simulink model "simulation_model"  (R2025a)
settings: Solver=ode4  StartTime=0.0  StopTime=1500  FixedStep=0.5  RelTol=1e-3
InitFcn:
  | init
StopFcn:
  | post_processing
values from neighbouring files (symbols this model uses):
  A0 = deg2rad(A0)    [init.m]
  delta0 = deg2rad(delta0)    [init.m]
  dT = 10    [init.m]
  fc = 0.62    [init.m]
  g = 9.80665    [init.m]
  Isp = zeros(1, 3)    [init.m]
  l_trilho = lt    (= 20.71)    [init.m]
  lc = 1.4    [init.m]
  lon0 = deg2rad(lon0)    [init.m]
  m0 = sum(mp) + sum(ms) + mL    [init.m]
  mp = zeros(1, 3)    [init.m]
  ms = zeros(1, 3)    [init.m]
  parametros_aero = [ts, Sr, fc]    [init.m]
  parametros_grav = [Re,mut,J2,J3,J4]    [init.m]
  phi0 = deg2rad(phi0)    [init.m]
  r0 = Re + h0    (= 6378137)    [init.m]
  Re = 6378.1370e3    (= 6378137)    [init.m]
  Sr = [S1, S2 * f2, S3 * f3, SL * f4]    [init.m]
  ti = zeros(1, 3)    [init.m]
  tq = zeros(1, 3)    [init.m]
  ts = zeros(1, 3)    [init.m]
  V0 = 7.2921150e-5    (= 7.292115e-05)    [init.m]
  we = 7.2921150e-5    (= 7.292115e-05)    [init.m]
settings Model: Creator=Guilherme  LastModifiedBy=Guilherme

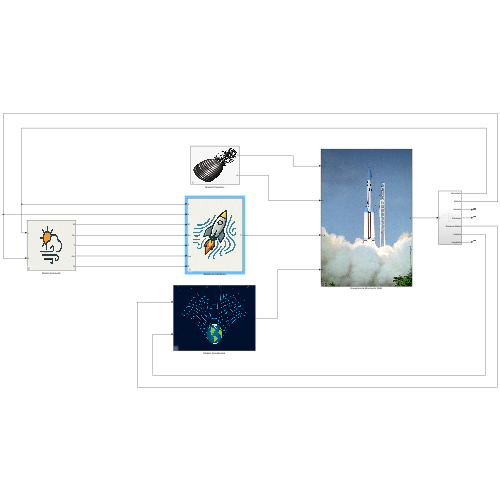
[thumbnail: Simulink's stored preview of the top-level diagram]
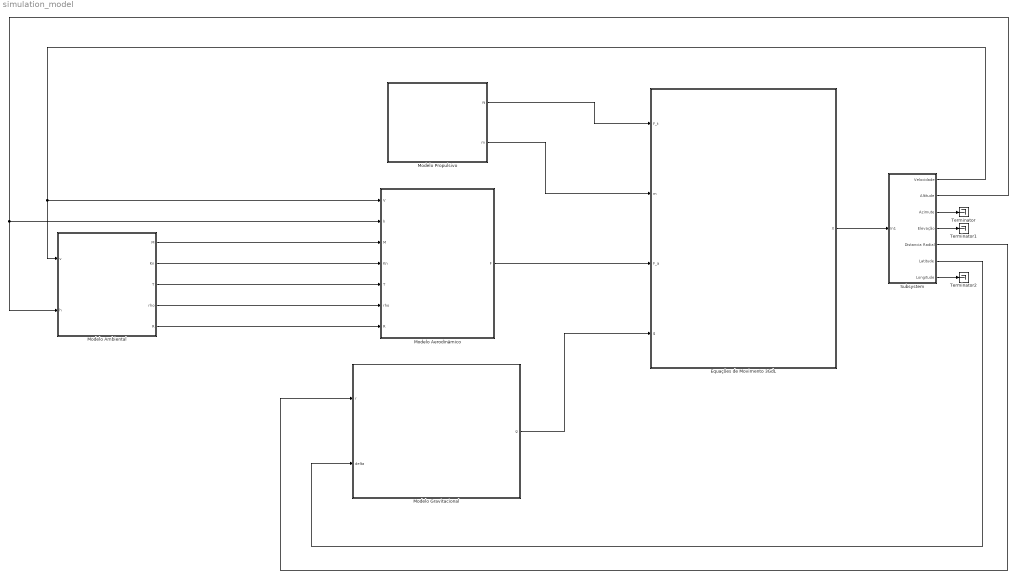
== system simulation_model ==
  Equações de Movimento 3GdL : Subsystem  mask{estado_inicial=[V0; A0; phi0; r0; delta0; lon0], trilho=l_trilho}
      mask prompts: estado_inicial "Vetor de estados inicial:"; trilho "Comprimeto do trilho de lançameto:"
      mask DialogControl texto Prompt: Bloco utilizado para simular as equações de movimento 3GdL de um foguete com 3 estágios. Os estados são organizados da seguinte forma:
      mask DialogControl Control2 Prompt: ● Magnitude da Velocidade - [m/s];
      mask DialogControl Control3 Prompt: ● Azimute Relativo - [rad];
      mask DialogControl Control4 Prompt: ● Ângulo de elevação da velocidade relativa - [rad];
      mask DialogControl Control5 Prompt: ● Distancia radial - [m];
      mask DialogControl Control6 Prompt: ● Latitude planetária - [rad];
      mask DialogControl Control7 Prompt: ● Longitude planetária - [rad].
      mask Display: image('EoM_mask.png');
  Modelo Aerodinâmico : Subsystem  mask{t_sep=ts, S_ref=Sr, fator_arrasto=fc}
      mask prompts: t_sep "Instante de separação dos estágios:"; S_ref "Vetor de áreas de referência:"; fator_arrasto "Fator de correção do arrasto:"
      mask DialogControl Control1 Prompt: Bloco utilizado para modelar a aerodinâmica do foguete. Calcula a força de arrasto a partir da velocidade e dos parâmetros atmosféricos. Os ângulos de ataque e derrapagem são assumidos zero.
      mask Display: image('aerodinamica_mask.png');
  Modelo Ambiental : Subsystem  mask{comprimento=lc, delta_T=dT}
      mask prompts: comprimento "Comprimento característico do veículo:"; delta_T "Variação de temperatura em relação à atmosfera padrão (15ºC no nível do mar):"
      mask DialogControl Control1 Prompt: Bloco utilizado para implementar o modelo de atmosfera padrão. Calcula os parâmetros atmosféricos com base na altitude de voo e velocidade.
      mask Display: image('atmosfera_mask.png');
  Modelo Gravitacional : Subsystem
      mask DialogControl Control1 Prompt: Bloco utilizado para implementar o modelo gravitacional do planeta Terra. Calcula as componentes centrípeta e radial da gravidade a partir da altitude e latitude do foguete.
      mask Display: image('gravidade_mask.png');
  Modelo Propulsivo : Subsystem  mask{t_ignicao=ti, t_queima=tq, t_sep=ts, massa_prop=mp, massa_est=ms, Isp_sub=Isp, massa0=m0}
      mask prompts: t_ignicao "Instantes de ignição:"; t_queima "Instantes do fim da queima:"; t_sep "Instantes de separação:"; massa_prop "Massa de propelente de cada eságio:"; massa_est "Massa estrutural de cada estágio:"; Isp_sub "Impulso específico de cada estágio:"; massa0 "Massa inicial do foguete:"
      mask DialogControl Control1 Prompt: Bloco utilizado por simular o efeito do sistema propulsivo do foguete. Calcula a força de tração e a massa do veículo a partir do estágio que está operando em cada instante de tempo.
      mask Display: image('motor_mask.jpg');
  Subsystem : Subsystem
  Terminator : Terminator
  Terminator1 : Terminator
  Terminator2 : Terminator
  wires:
  Modelo Propulsivo/1(ft) -> Equações de Movimento 3GdL/1(F_t)
  Modelo Propulsivo/2(m) -> Equações de Movimento 3GdL/2(m)
  Modelo Aerodinâmico/1(F) -> Equações de Movimento 3GdL/3(F_a)
  Modelo Ambiental/1(M) -> Modelo Aerodinâmico/3(M)
  Modelo Ambiental/2(Kn) -> Modelo Aerodinâmico/4(Kn)
  Modelo Ambiental/3(T) -> Modelo Aerodinâmico/5(T)
  Modelo Ambiental/4(rho) -> Modelo Aerodinâmico/6(rho)
  Modelo Ambiental/5(R) -> Modelo Aerodinâmico/7(R)
  Modelo Gravitacional/1(g) -> Equações de Movimento 3GdL/4(g)
  Equações de Movimento 3GdL/1(X) -> Subsystem/1(In1)
  Subsystem/1(Velocidade) -> Modelo Ambiental/1(v), Modelo Aerodinâmico/1(V)
  Subsystem/2(Altitude) -> Modelo Aerodinâmico/2(h), Modelo Ambiental/2(h)
  Subsystem/5(Distancia Radial) -> Modelo Gravitacional/1(r)
  Subsystem/3(Azimute) -> Terminator/1
  Subsystem/4(Elevação) -> Terminator1/1
  Subsystem/7(Longitude) -> Terminator2/1
  Subsystem/6(Latitude) -> Modelo Gravitacional/2(delta)

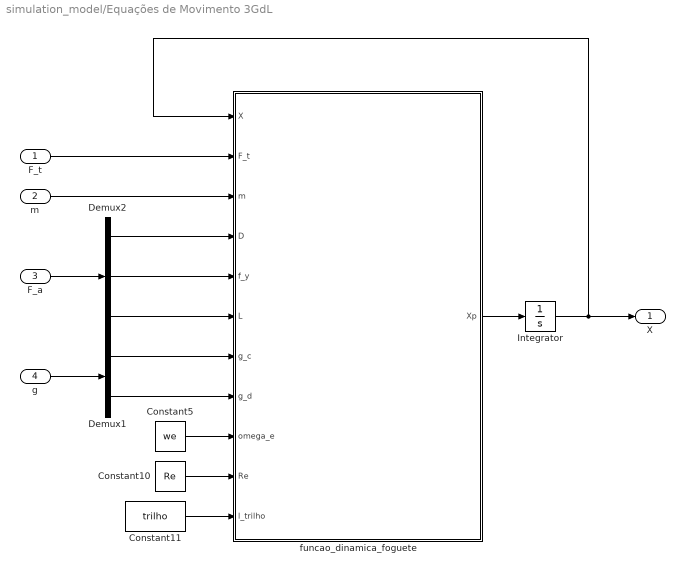
== system simulation_model/Equações de Movimento 3GdL ==
  F_t : Inport
  m : Inport  Port=2
  F_a : Inport  Port=3
  g : Inport  Port=4
  Constant10 : Constant  Value=Re
  Constant11 : Constant  Value=trilho
  Constant5 : Constant  Value=we
  Demux1 : Demux  Outputs=2
  Demux2 : Demux  Outputs=3
  Integrator : Integrator  InitialCondition=estado_inicial
  funcao_dinamica_foguete : MATLAB Function  TreatAsAtomicUnit=on
  X : Outport
  wires:
  Demux2/1 -> funcao_dinamica_foguete/4(D)
  funcao_dinamica_foguete/1(Xp) -> Integrator/1
  Constant5/1 -> funcao_dinamica_foguete/9(omega_e)
  Integrator/1 -> X/1, funcao_dinamica_foguete/1(X)
  Constant10/1 -> funcao_dinamica_foguete/10(Re)
  Demux2/3 -> funcao_dinamica_foguete/6(L)
  F_t/1 -> funcao_dinamica_foguete/2(F_t)
  g/1 -> Demux1/1
  Constant11/1 -> funcao_dinamica_foguete/11(l_trilho)
  Demux1/1 -> funcao_dinamica_foguete/7(g_c)
  Demux2/2 -> funcao_dinamica_foguete/5(f_y)
  Demux1/2 -> funcao_dinamica_foguete/8(g_d)
  m/1 -> funcao_dinamica_foguete/3(m)
  F_a/1 -> Demux2/1

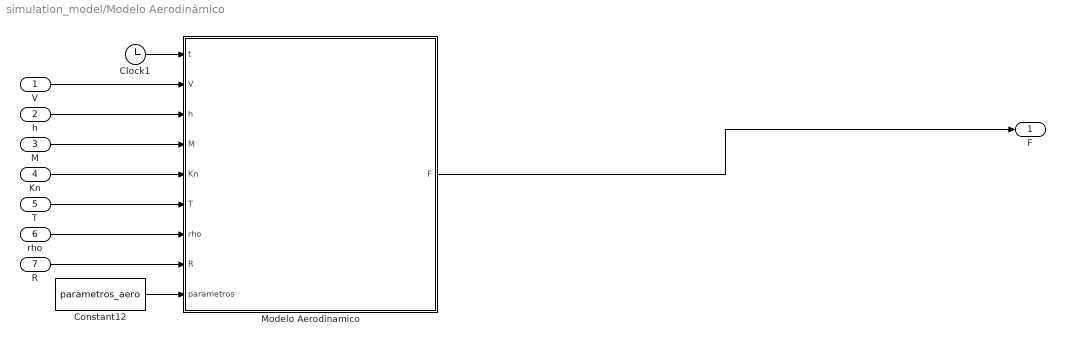
== system simulation_model/Modelo Aerodinâmico ==
  V : Inport
  h : Inport  Port=2
  M : Inport  Port=3
  Kn : Inport  Port=4
  T : Inport  Port=5
  rho : Inport  Port=6
  R : Inport  Port=7
  Clock1 : Clock
  Constant12 : Constant  Value=parametros_aero
  Modelo Aerodinamico : MATLAB Function  TreatAsAtomicUnit=on
  F : Outport
  wires:
  Constant12/1 -> Modelo Aerodinamico/9(parametros)
  M/1 -> Modelo Aerodinamico/4(M)
  Modelo Aerodinamico/1(F) -> F/1
  R/1 -> Modelo Aerodinamico/8(R)
  h/1 -> Modelo Aerodinamico/3(h)
  V/1 -> Modelo Aerodinamico/2(V)
  Clock1/1 -> Modelo Aerodinamico/1(t)
  T/1 -> Modelo Aerodinamico/6(T)
  Kn/1 -> Modelo Aerodinamico/5(Kn)
  rho/1 -> Modelo Aerodinamico/7(rho)

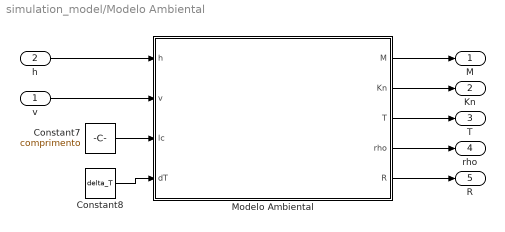
== system simulation_model/Modelo Ambiental ==
  v : Inport
  h : Inport  Port=2
  Constant7 : Constant  Value=comprimento
  Constant8 : Constant  Value=delta_T
  Modelo Ambiental : MATLAB Function  TreatAsAtomicUnit=on
  M : Outport
  Kn : Outport  Port=2
  T : Outport  Port=3
  rho : Outport  Port=4
  R : Outport  Port=5
  wires:
  Modelo Ambiental/2(Kn) -> Kn/1
  Constant7/1 -> Modelo Ambiental/3(lc)
  Modelo Ambiental/3(T) -> T/1
  Constant8/1 -> Modelo Ambiental/4(dT)
  Modelo Ambiental/1(M) -> M/1
  h/1 -> Modelo Ambiental/1(h)
  Modelo Ambiental/4(rho) -> rho/1
  Modelo Ambiental/5(R) -> R/1
  v/1 -> Modelo Ambiental/2(v)

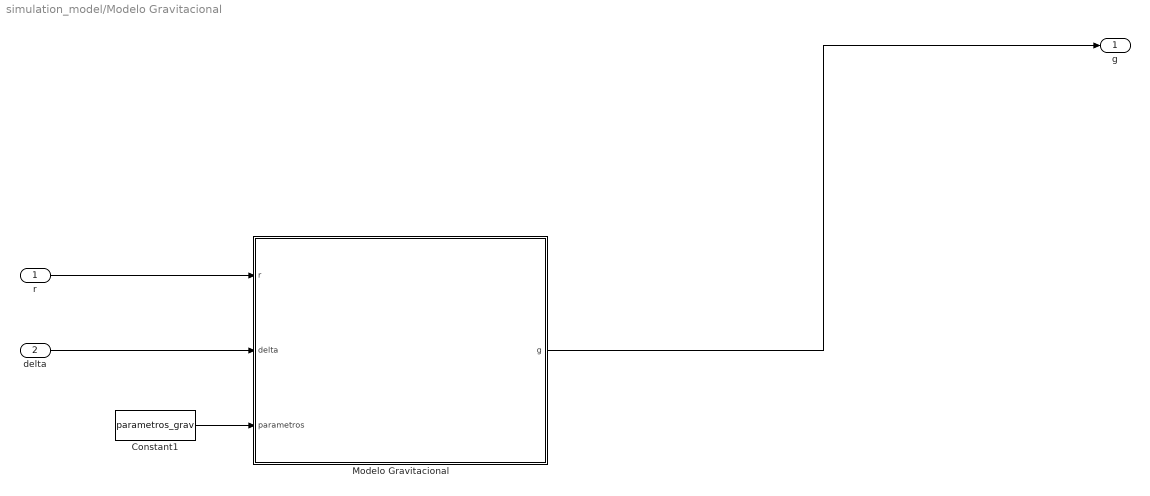
== system simulation_model/Modelo Gravitacional ==
  r : Inport
  delta : Inport  Port=2
  Constant1 : Constant  Value=parametros_grav
  Modelo Gravitacional : MATLAB Function  TreatAsAtomicUnit=on
  g : Outport
  wires:
  Constant1/1 -> Modelo Gravitacional/3(parametros)
  delta/1 -> Modelo Gravitacional/2(delta)
  r/1 -> Modelo Gravitacional/1(r)
  Modelo Gravitacional/1(g) -> g/1

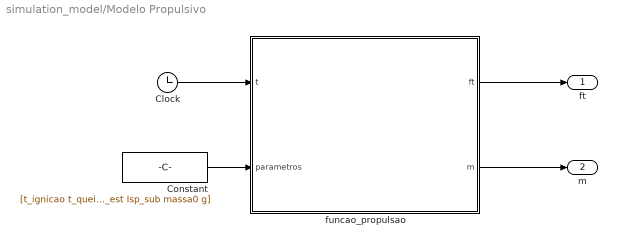
== system simulation_model/Modelo Propulsivo ==
  Clock : Clock
  Constant : Constant  Value=[t_ignicao t_queima t_sep massa_prop massa_est Isp_sub massa0 g]
  funcao_propulsao : MATLAB Function  TreatAsAtomicUnit=on
  ft : Outport
  m : Outport  Port=2
  wires:
  Clock/1 -> funcao_propulsao/1(t)
  Constant/1 -> funcao_propulsao/2(parametros)
  funcao_propulsao/1(ft) -> ft/1
  funcao_propulsao/2(m) -> m/1

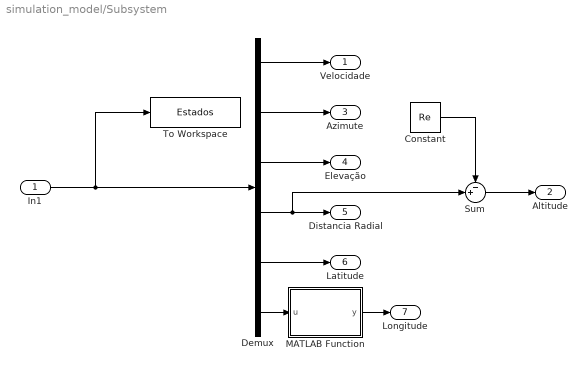
== system simulation_model/Subsystem ==
  In1 : Inport
  Constant : Constant  Value=Re
  Demux : Demux  Outputs=6
  MATLAB Function : MATLAB Function  TreatAsAtomicUnit=on
  Sum : Sum  Inputs=-+|
  To Workspace : ToWorkspace  VariableName=Estados  SampleTime=-1
      settings: Save2DSignal=2-D array (concatenate along first dimension)
  Velocidade : Outport
  Altitude : Outport  Port=2
  Azimute : Outport  Port=3
  Elevação : Outport  Port=4
  Distancia Radial : Outport  Port=5
  Latitude : Outport  Port=6
  Longitude : Outport  Port=7
  wires:
  Demux/1 -> Velocidade/1
  In1/1 -> To Workspace/1, Demux/1
  Demux/6 -> MATLAB Function/1(u)
  Demux/4 -> Sum/2, Distancia Radial/1
  MATLAB Function/1(y) -> Longitude/1
  Demux/5 -> Latitude/1
  Demux/2 -> Azimute/1
  Demux/3 -> Elevação/1
  Constant/1 -> Sum/1
  Sum/1 -> Altitude/1

== matlab function simulation_model/Modelo Propulsivo/funcao_propulsao ==
  data: t input; ft output; parametros input; m output
function [ft, m] = propulsor_3_estagios(t, parametros)
    % Modelo de propulsor de foguete de 3 estágios
    % Entradas:
    % t          - Tempo atual
    % parametros - Vetor contendo os parâmetros do modelo:
    %   parametros(1:3)  - Tempos de ignição (ti)
    %   parametros(4:6)  - Tempos de queima contínua (tq)
    %   parametros(7:9)  - Tempos de separação (ts)
    %   parametros(10:12)- Massa de propelente (mp)
    %   parametros(13:15)- Massa de separação (ms)
    %   parametros(16)   - Massa inicial (m0)
    %   parametros(17)   - Gravidade (g)
    
    % Extração dos parâmetros do vetor
    ti = parametros(1:3);         % Tempos de ignição
    tq = parametros(4:6);         % Tempos de queima contínua
    ts = parametros(7:9);         % Tempos de separação
    mp = parametros(10:12);       % Massas de propelente
    ms = parametros(13:15);       % Massas de separação
    Isp = parametros(16:18);      % Impulsos específicos
    m0 = parametros(19);          % Massa inicial
    g = parametros(20);           % Gravidade
    
    % Função de cálculo da força propulsiva e da massa para cada estágio
    if t <= ti(1)
        % Antes da ignição do primeiro estágio
        m = m0;
        ft = 0;
    elseif t <= tq(1)
        % Durante a queima contínua do primeiro estágio
        md = -mp(1) / (tq(1) - ti(1));  % Taxa de queima
        m = m0 + md * (t - ti(1));      % Massa durante a queima
        ft = -g * Isp(1) * md;          % Força propulsiva do primeiro estágio
    elseif t <= ts(1)
        % Após a queima do primeiro estágio e antes da separação
        m = m0 - mp(1);
        ft = 0;
    elseif t <= ti(2)
        % Entre a separação do primeiro estágio e a ignição do segundo
        m = m0 - mp(1) - ms(1);
        ft = 0;
    elseif t <= tq(2)
        % Durante a queima contínua do segundo estágio
        md = -mp(2) / (tq(2) - ti(2));  % Taxa de queima do segundo estágio
        m02 = m0 - mp(1) - ms(1);       % Massa inicial para o segundo estágio
        m = m02 + md * (t - ti(2));     % Massa durante a queima
        ft = -g * Isp(2) * md;          % Força propulsiva do segundo estágio
    elseif t <= ts(2)
        % Após a queima do segundo estágio e antes da separação
        m = m0 - mp(1) - ms(1) - mp(2);
        ft = 0;
    elseif t <= ti(3)
        % Entre a separação do segundo estágio e a ignição do terceiro
        m = m0 - mp(1) - ms(1) - mp(2) - ms(2);
        ft = 0;
    elseif t <= tq(3)
        % Durante a queima contínua do terceiro estágio
        md = -mp(3) / (tq(3) - ti(3));  % Taxa de queima do terceiro estágio
        m03 = m0 - mp(1) - ms(1) - mp(2) - ms(2);  % Massa inicial para o terceiro estágio
        m = m03 + md * (t - ti(3));     % Massa durante a queima
        ft = -g * Isp(3) * md;          % Força propulsiva do terceiro estágio
    elseif t <= ts(3)
        % Após a queima do terceiro estágio e antes da separação
        m = m0 - mp(1) - ms(1) - mp(2) - ms(2) - mp(3);
        ft = 0;
    else
        % Após a separação do terceiro estágio
        m = m0 - mp(1) - ms(1) - mp(2) - ms(2) - mp(3) - ms(3);
        ft = 0;
    end
end

== matlab function simulation_model/Equações de Movimento 3GdL/funcao_dinamica_foguete ==
  data: X input; Xp output; F_t input; m input; D input; f_y input; L input; g_c input; g_d input; omega_e input; Re input; l_trilho input
function Xp = dinamica_foguete(X, F_t, m, D, f_y, L, g_c, g_d, omega_e,Re,l_trilho)
    % Função para a dinâmica de translação de um foguete com respeito ao referencial PCPF
    % Sistema de referência: aerodinâmico
    % Sistema de coordenadas: esférico
    
    % Vetor de estado
    V = X(1);    % Velocidade
    A = X(2);    % Ângulo de azimute
    phi = X(3);  % Ângulo de elevação
    r = X(4);    % Distância radial
    delta = X(5); % Latitude
    lon = X(6);   % Longitude
    h = r - Re;   % Altitude

    % Equações de cinemática de translação
    rp = V * sin(phi);
    deltap = (V / r) * cos(phi) * cos(A);
    lonp = (V * cos(phi) * sin(A)) / (r * cos(delta));

    % Equações de dinâmica de translação
    Vp = (1 / m) * (F_t * cos(0) * cos(0) - D - m * g_c * sin(phi) + m * g_d * cos(phi) * cos(A) - ... 
        m * omega_e^2 * r * cos(delta) * (cos(phi) * cos(A) * sin(delta) - sin(phi) * cos(delta)));
    
    Ap = (1 / (m * V * cos(phi))) * (m * (V^2 / r) * cos(phi)^2 * sin(A) * tan(delta) + F_t * sin(0) + ... 
        f_y - m * g_d * sin(A) + m * omega_e^2 * r * sin(A) * sin(delta) * cos(delta) - ... 
        2 * m * omega_e * V * (sin(phi) * cos(A) * cos(delta) - cos(phi) * sin(delta)));

    phip = (1 / (m * V)) * (m * (V^2 / r) * cos(phi) + F_t * sin(0) * cos(0) + L - m * g_c * cos(phi) - ... 
        m * g_d * sin(phi) * cos(A) + m * omega_e^2 * r * cos(delta) * (sin(phi) * cos(A) * sin(delta) + ... 
        cos(phi) * cos(delta)) + 2 * m * omega_e * V * sin(A) * cos(delta));
    
    % Saturação da altitude
    if h < 0  % Altitude negativa não é permitida
        % Mantém as derivadas nulas
        rp = 0; deltap = 0; lonp = 0; Ap = 0; phip = 0;
    end

    % Modela o trilho de lançamento
    if h <= l_trilho  % Verifica se a altura é menor que l_trilho nos primeiros segundos da simulação
        Ap = 0; phip = 0;  % Anula as derivadas dos ângulos de orientação da velocidade
    end
    
    % Derivadas dos estados
    Xp = [Vp; Ap; phip; rp; deltap; lonp];
end

== matlab function simulation_model/Modelo Ambiental/Modelo Ambiental ==
  data: h input; v input; lc input; dT input; M output; Kn output; T output; rho output; R output
function [M, Kn, T, rho, R] = atm_padrao(h, v, lc, dT)
    % Função para calcular as propriedades atmosféricas com base na altitude
    % h: Altitude geométrica (m)
    % v: Velocidade do veículo (m/s)
    % lc: Comprimento característico do veículo (m)
    % dT: Variação de temperatura em relação à temperatura padrão (K ou °C)
    
    % Dados do modelo de atmosfera (altitudes em metros)
    hi = [0, 11.0191, 20.0631, 32.1619, 47.3501, 51.4125, 71.8020, 86, 100, 110, 120, 150, ...
          160, 170, 190, 230, 300, 400, 500, 600, 700] * 1e3;  % km convertido para metros
    Ti = [288.15, 216.65, 216.65, 228.65, 270.65, 270.65, 214.65, 186.946, 210.65, 260.65, 360.65, ...
          960.65, 1110.65, 1210.65, 1350.65, 1550.65, 1830.65, 2160.65, 2420.65, 2590.65, 2700.65];
    Ri = [287.0, 287.0, 287.0, 287.0, 287.0, 287.0, 287.02, 287.02, 287.84, 291.06, 308.79, 311.80, ...
          313.69, 321.57, 336.68, 366.84, 416.88, 463.36, 493.63, 514.08, 514.08];
    a = [-6.5, 0.0, 1.0, 2.8, 0.0, -2.8, -2.0, 1.693, 5.0, 10.0, 20.0, 15.0, 10.0, 7.0, 5.0, ...
         4.0, 3.3, 2.6, 1.7, 1.1, 0.0] * 1e-3;  % °/m
    Mi = [28.9644, 28.9644, 28.9644, 28.9644, 28.9644, 28.9644, 28.9644, 28.9644, ...
          28.88, 28.56, 28.07, 26.92, 26.66, 26.4, 25.85, 24.7, 22.66, 19.94, 17.94, 16.84, 16.17];

    % Constantes
    M0 = Mi(1);  % Peso molecular ao nível do mar
    g0 = 9.80665;  % Aceleração da gravidade (m/s²)
    Na = 6.0220978e23;  % Número de Avogadro
    sigma = 3.65e-10;  % Diâmetro de colisão para o ar (m)
    m0 = 28.964e-3;  % Massa molar do ar ao nível do mar (kg/mol)
    P0 = 1.01325e5;  % Pressão padrão ao nível do mar (N/m²)
    Re = 6378.14e3;  % Raio médio da Terra (m)
    gamma = 1.405;  % Razão de calores específicos ao nível do mar
    
    % Constantes calculadas
    beta = 2 / Re;  % Número beta associado à distância radial média do nível do mar
    
    % Identifica a camada a qual a altitude pertence
    if h < 0
        % Altitude negativa. Ajusta para h=0.
        i = 1;
        h = 0;
    elseif h > 2000e3
        % Altitude acima de 2000 km. Ajusta para h=2000 km.
        i = 20;
        h = 2000e3;
    else
        for i = 1:21
            if i == 20
                break
            elseif h >= hi(i) && h < hi(i + 1)
                break
            end
        end
    end
    
    % Calcula a pressão no início da camada i
    Pi = P0;
    px = P0;  % Variável auxiliar para guardar o valor de pressão inicial na camada anterior
    for j = 2:i
        if a(j-1) ~= 0
            % Se a camada não for isotérmica
            A = 1 + (a(j-1) * (hi(j) - hi(j-1))) / Ti(j-1);
            B = -(g0 / (Ri(j) * a(j-1))) * (1 + beta * (Ti(j-1) / a(j-1) - hi(j-1)));
            C = (g0 * beta / (Ri(j) * a(j-1))) * (hi(j) - hi(j-1));
            Pi = px * (A^B) * exp(C);
            px = Pi;  % Atualiza o valor de px
        else
            % Camada isotérmica
            Pi = px * exp(-(g0 / (Ri(j) * Ti(j-1))) * (hi(j) - hi(j-1)) * (1 - (beta / 2) * (hi(j) - hi(j-1))));
            px = Pi;
        end
    end
    
    % Temperatura padrão (molecular) usada nos cálculos internos
    Tm = Ti(i) + a(i) * (h - hi(i));
    
    % Corrige pelo valor de delta T adotado
    Tm = Tm + dT;
    
    % Interpola o valor de R e M
    if i >= 20
        R = Ri(i);
        M = Mi(i);
    else
        R = Ri(i) + ((Ri(i + 1) - Ri(i)) / (hi(i + 1) - hi(i))) * (h - hi(i));
        M = Mi(i) + ((Mi(i + 1) - Mi(i)) / (hi(i + 1) - hi(i))) * (h - hi(i));
    end
    
    % Temperatura padrão (cinética) - saída da função
    T = (M / M0) * Tm;
    
    % Calcula a pressão
    if a(i) ~= 0
        A = 1 + (a(i) * (h - hi(i))) / Ti(i);
        B = -(g0 / (R * a(i))) * (1 + beta * (Ti(i) / a(i) - hi(i)));
        C = (g0 * beta / (R * a(i))) * (h - hi(i));
        p = Pi * (A^B) * exp(C);
    else
        p = Pi * exp(-(g0 / (R * Ti(i))) * (h - hi(i)) * (1 - (beta / 2) * (h - hi(i))));
    end
    
    % Calcula a densidade
    rho = p / (R * Tm);
    
    % Velocidade do som
    ainf = sqrt(gamma * R * Tm);
    
    % Número de Mach
    M = v / ainf;
    
    % Coeficiente de viscosidade dinâmica
    mu = 1.458e-6 * (Tm^(3 / 2)) / (Tm + 110.4);
    
    % Número de Prandtl
    cp = R * gamma / (gamma - 1);
    kT = (2.64638e-3 * (Tm^(3 / 2))) / (Tm + 245.4 * (10^(-12 / Tm)));
    Pr = mu * cp / kT;
    
    % Número de Knudsen
    lam = m0 / (sqrt(2) * pi * sigma^2 * rho * Na);
    Kn = lam / lc;
    
    % Parâmetro de regime de escoamento
    if Kn >= 10
        d = 1;
    elseif Kn <= 0.01
        d = 2;
    else
        d = 3;
    end
    
    % Número de Reynolds
    Re = rho * v * lc / mu;
end

== matlab function simulation_model/Modelo Aerodinâmico/Modelo Aerodinamico ==
  data: t input; V input; h input; M input; F output; Kn input; T input; rho input; R input; parametros input
% Função principal de arrasto para 3 estágios
function F = aerodinamica_3_estagios(t, V, h, M, Kn, T, rho, R,parametros)
    % Modelo de arrasto conforme a referência de Tewari, 2007
    % Assume-se o mesmo coeficiente de arrasto para o foguete e seus estágios
    
    % Variáveis globais do parâmetro de simulação (parametros)
    ts = parametros(1:3);
    Sr = parametros(4:7);
    fc = parametros(8);
    
    % Coeficiente de arrasto em função do número de Mach e de Knudsen
    CD = coefArrastoFoguete(V, h, M, Kn, T, R);
    
    % Fator de correção do arrasto a partir de dados de túnel de vento
    CD = fc * CD;
    
    % A área de referência depende do estágio atual
    S = area3estagios(t, ts, Sr);
    
    % Cálculo da força de arrasto
    D = 0.5 * rho * V^2 * S * CD;
    
    % Forças laterais e de sustentação (supondo zero neste exemplo)
    fy = 0;
    L = 0;
    F = [D fy L];

function CDc = iterpCD(M)
    % Dados extraídos de Tewari
    CD_data = [4.44e-16, 0.47;
          0.16, 0.47; 0.34, 0.48; 0.48, 0.49; 0.53, 0.50; 0.64, 0.51; 0.71, 0.54;
          0.75, 0.56; 0.85, 0.59; 0.87, 0.62; 0.91, 0.67; 0.94, 0.64; 0.95, 0.70;
          0.95, 0.72; 0.97, 0.79; 0.98, 0.80; 0.99, 0.87; 1.0, 0.89; 1.01, 1.03;
          1.011, 0.98; 1.018, 0.95; 1.025, 1.013; 1.034, 0.97; 1.13, 1.013;
          1.15, 1.0; 1.22, 0.98; 1.26, 0.97; 1.27, 0.96; 1.30, 0.94; 1.35, 0.92;
          1.40, 0.90; 1.44, 0.88; 1.49, 0.86; 1.53, 0.84; 1.58, 0.82; 1.67, 0.79;
          1.74, 0.77; 1.81, 0.75; 1.88, 0.73; 1.98, 0.70; 2.18, 0.66; 2.28, 0.64;
          2.36, 0.63; 2.61, 0.59; 2.73, 0.58; 2.87, 0.56; 2.99, 0.55; 3.17, 0.54;
          3.43, 0.53; 3.68, 0.52; 3.97, 0.51; 4.18, 0.51; 4.44, 0.50; 4.69, 0.50;
          4.95, 0.49; 5.18, 0.49; 5.44, 0.49; 5.69, 0.49; 5.95, 0.49; 6.20, 0.49;
          6.45, 0.49; 6.70, 0.49; 6.95, 0.49; 7.20, 0.49; 7.46, 0.49; 7.71, 0.49;
          7.96, 0.49; 8.21, 0.49; 8.46, 0.49; 8.71, 0.49; 8.97, 0.48; 9.22, 0.48;
          9.47, 0.48; 9.72, 0.48; 10.22, 0.48; 10.47, 0.48; 10.73, 0.48;
          10.98, 0.48; 11.23, 0.48; 11.48, 0.48; 11.73, 0.48];

    % Remover valores duplicados na primeira coluna
    [~, ia, ~] = unique(CD_data(:, 1), 'first');
    CD_data = CD_data(ia, :); % Filtra os valores duplicados

    % Interpolação para o número de Mach da entrada
    f = @(M) interp1(CD_data(:,1), CD_data(:,2), M, 'linear', 'extrap');
    
    % Evita erro de interpolação
    if M <= 0
        M = 0;
    elseif M > 11.73
        M = 11.73;
    end
    
    % Calcular CDc
    CDc = f(M);
end

% Função para calcular o coeficiente de arrasto do foguete
function CD = coefArrastoFoguete(V, h, M, Kn, T, R)
    % Calcula o coeficiente de arrasto para o foguete
    
    if V ~= 0
        s = V / sqrt(2 * R * T);
    else
        s = 1E-16 / sqrt(2 * R * T);
    end
    
    CDfm = 1.75 + sqrt(pi) / (2 * s);
    CDc = iterpCD(M);
    
    if h < 2000e3
        if Kn < 0.0146  % Meio contínuo
            CD = CDc;
        elseif Kn < 14.5  % Transição entre o contínuo e o livre molecular
            CD = CDc + (CDfm - CDc) * ((1 / 3) * log10(Kn / sin(30 * pi / 180)) + 0.5113);
        else  % Escoamento livre molecular
            CD = CDfm;
        end
    else  % Sem arrasto
        CD = 0;
    end
end

function S = area3estagios(t, ts, Sr)
    % Função para determinar a área de referência do arrasto em função do tempo
    % t: Tempo atual
    % ts: Vetor com os tempos de separação dos estágios (3 elementos)
    % Sr: Vetor com as áreas de referência dos estágios e da carga útil (4 elementos)

    if t <= ts(1)
        % Todos os estágios
        S = Sr(1);
    elseif t <= ts(2)
        % Segundo estágio
        S = Sr(2);
    elseif t <= ts(3)
        % Terceiro estágio e carga útil
        S = Sr(3);
    else
        % Apenas a carga útil
        S = Sr(4);
    end
end

end

== matlab function simulation_model/Modelo Gravitacional/Modelo Gravitacional ==
  data: r input; g output; delta input; parametros input
function g = grav_axisimetrico(r, delta, parametros)
    % Função para calcular as componentes da gravidade no modelo gravitacional axissimétrico
    % Entradas:
    % r: Distância radial ao centro de massa do planeta (m)
    % delta: Latitude centrada no planeta (rad)
    % parametros: Estrutura contendo os parâmetros do modelo (RE, MU, J2, J3, J4)
    
    % Extração dos parâmetros da estrutura de entrada
    Re = parametros(1);   % Raio médio da Terra (m)
    mu = parametros(2);   % Constante gravitacional da Terra (m^3/s^2)
    J2 = parametros(3);   % Parâmetro J2
    J3 = parametros(4);   % Parâmetro J3
    J4 = parametros(5);   % Parâmetro J4

    % Colatitude (rad)
    phi = pi / 2 - delta; 
    
    % Componente radial da gravidade de corpo axissimétrico
    gr = (1 / r^6) * mu * (-r^4 - 1.5 * J2 * r^2 * Re^2 + 1.875 * J4 * Re^4 - 6 * J3 * r * Re^3 * cos(phi) + ...
        (4.5 * J2 * r^2 * Re^2 - 18.75 * J4 * Re^4) * cos(phi)^2 + 10 * J3 * r * Re^3 * cos(phi)^3 + ...
        21.875 * J4 * Re^4 * cos(phi)^4);
    
    % Componente sul (direção phi) da gravidade de corpo axissimétrico
    gphi = (1 / r^6) * 3 * mu * Re^2 * (-0.5 * J3 * r * Re + (J2 * r^2 - 2.5 * J4 * Re^2) * cos(phi) + ...
        2.5 * J3 * r * Re * cos(phi)^2 + 5.83333 * J4 * Re^2 * cos(phi)^3) * sin(phi);

    % Componentes nas direções centrípeta e latitudinal (norte)
    gc = -gr;  % Componente centrípeta da gravidade
    gdel = -gphi;  % Componente latitudinal da gravidade
    
    g = [gc gdel];
end

== matlab function simulation_model/Subsystem/MATLAB Function ==
  data: u input; y output
function y = fcn(u)

y = wrapToPi(u);
